simulink model "Studienarbeit"  (R2020a)
settings: Solver=VariableStepAuto  StartTime=0.0  StopTime=300  FixedStep=0.1  RelTol=1e-3
values from neighbouring files (symbols this model uses):
  driver_I = 0.1    [Buses_.mat]    (also in helperACCSetUp.m)
  driver_P = 0.2    [Buses_.mat]    (also in helperACCSetUp.m)
  initial_lane = 0    [helperACCSetUp.m]
  lr = 1.6    [Buses_.mat]    (also in helperACCSetUp.m)
  m = 1575    [Buses_.mat]    (also in helperACCSetUp.m)
  tau = 0.5    [Buses_.mat]    (also in helperACCSetUp.m)
  velocity_left_lane_max = 28    [Buses_.mat]    (also in helperManeuverSetUp.m)
  velocity_right_lane_max = 20    [Buses_.mat]    (also in helperManeuverSetUp.m)
  velocity_vehicle_B = 10    [Buses_.mat]    (also in helperManeuverSetUp.m)
  yawerr_gain = 2    [Buses_.mat]    (also in helperACCSetUp.m)
undefined symbols (not defined in the file or in its folder): Curvature, CurvatureDerivative, driving, HeadingAngle, LateralOffset, Left, Right, Strength
libraries: drivingscenarioandsensors x3, simulink x1, autolibshared x1
(part 2 of 2)

== matlab function Studienarbeit/Vehicle and Environment and Maneuver/Actors and Sensor Simulation/Pack Ego Actor ==
  data: pos input; egoActor output Bus: BusActors1Actors size=1; vel input; yaw input; yawRate input
function egoActor = packEgo(pos,vel,yaw,yawRate)
% Pack ego information into a single ego actor bus
%
% Imoprtant note:
% Output is a bus of type BusActorsActors. This is the same bus used by the
% Scenario Reader to output an individual actor. If you change the
% output bus name of Scenario Reader, change the output bus name here
% as well by clicking on 'Edit Data' in the menu above.
% if pos(2)<=-2
%     pos(2)=-2;
% elseif pos(2)>=2
%     pos(2)=2;
% end

egoActor = struct(...
    'ActorID',1,...
    'Position', [pos(1) pos(2) 0], ...
    'Velocity', [vel(1) vel(2) 0], ...
    'Roll', 0, ...
    'Pitch', 0, ...
    'Yaw', yaw, ...
    'AngularVelocity', [0 0 yawRate]);

== matlab function Studienarbeit/Vehicle and Environment and Maneuver/Control Unit/Steering Angle decide/Curve Lane or Not ==
  data: steeringLKA input; curve_lane_or_not output
function curve_lane_or_not = is_curve_lane(steeringLKA)
% This function uses steering angle from LKA to judge whether the lane 
% curve is,so that the vehicle will use another algorithm to achieve curve 
% lane changing.

% Input:
% steeringLKA: steering angle from Lane Keeping Assist.

% Output:
% curve_lane_or_not: 0->not a curve lane,1->curve lane.

if abs(steeringLKA) >10^(-2.5)%(-2.8)
    curve_lane_or_not = 1;
else
    curve_lane_or_not = 0;
end
% if abs(steeringLKA) >10^(-3)||(abs(Curvature_1)>10^(-4)||abs(Curvature_)>10^(-4))
%     curve_lane_or_not = 1;
% else
%     curve_lane_or_not = 0;
% end

== matlab function Studienarbeit/Vehicle and Environment and Maneuver/Control Unit/Steering Angle decide/Yaw Angle Process ==
  data: yaw_angle_ori input; yaw_angle output; curve_lane_or_not input
function yaw_angle = yaw_angle_process(yaw_angle_ori, curve_lane_or_not)
% This function subtracts a multiple of pi/2 rad from yaw angle when the 
% lane is straight,so that the vehicle can change its lane in straight lane 
% with a yaw angle larger than pi/2 rad.

% Inputs:
% yaw_angle_ori: original yaw angle(before processing).
% curve_lane_or_not: 0->not a curve lane,1->curve lane.

% Output:
% yaw_angle: the yaw angle after processing.

if curve_lane_or_not == 0
    yaw_angle=yaw_angle_ori-sign(yaw_angle_ori)*pi/2*round(abs(yaw_angle_ori)*2/pi);    
else 
    yaw_angle=yaw_angle_ori;
end

== stateflow chart Studienarbeit/Vehicle and Environment and Maneuver/Control Unit/Vehicle States ==
  state left_u_turn
    state decelerate
      entry:
      turn_flag = 5;
      coor_trans_t = clock_time;
      initial_lane_changing_velocity_ego = longitudinal_velocity;
    state turn_left
      entry:
      turn_flag = 6;
    state turn_left_1
      entry:
      turn_flag = 9;
    state backwards
      entry:
      turn_flag = 7;
    state turn_left_a_little
      entry:
      turn_flag = 8;
    decelerate -> turn_left : after(duration_lane_changing,sec)
    turn_left -> backwards : after(duration_lane_changing,sec)
    backwards -> turn_left_a_little : after(duration_lane_changing,sec)
    turn_left_a_little -> turn_left_1 : after(duration_lane_changing,sec)
  state switch_left_curve
    entry:
    turn_flag = 3;
  state switch_left
    entry:
    turn_flag = 1;
    coor_trans_t = clock_time;
    initial_lane_changing_velocity_ego = longitudinal_velocity;
  state lane_keeping
    entry:
    turn_flag = 0;
  state switch_right
    entry:
    turn_flag = 2;
    coor_trans_t = clock_time;
    initial_lane_changing_velocity_ego = longitudinal_velocity;
  state switch_right_curve
    entry:
    turn_flag = 4;
  note: command = 1, the vehicle switchs left,and turn_flag = 1.
      | command = 2, the vehicle switchs right,and turn_flag = 2.
      | if vehicle keeps lane, turn_flag = 0.
      | coor_trans_t is a time value which is used for coordinate transformation in
      | next subsystem:
      | "Duration,Curvature and Longitudinal Acceleration calculation".
      | initial_velocity_ego is the initial speed for the different maneuver.
      | current_lane = 0, the vehicle is at right lane.
      | current_lane = 1, the vehicle is at left lane
      | curve_lane_or_not = 0: the vehicle is driving at a curve lane.
      | curve_lane_or_not = 1: the vehicle is driving at a straight lane.
  lane_keeping -> decelerate [order 5] : [command == 5]
  lane_keeping -> switch_left_curve [order 3] : [command == 3]
  switch_left_curve -> lane_keeping : [left_boundary_strength>0.45&&right_boundary_strength< 0.15||left_lateral<0.22]{current_lane = 1;}
  (default) -> lane_keeping
  lane_keeping -> switch_left [order 2] : [command == 1]
  turn_left_1 -> lane_keeping : after(duration_lane_changing,sec){current_lane=1;}
  switch_left -> lane_keeping : after(duration_lane_changing,sec){current_lane = 1;}
  switch_right_curve -> lane_keeping : [left_boundary_strength<0.15&&right_boundary_strength >0.45||abs(right_lateral)<0.22]{current_lane = 0;}
  lane_keeping -> switch_right_curve [order 4] : [command==4]
  lane_keeping -> switch_right [order 1] : [command==2]
  switch_right -> lane_keeping : after(duration_lane_changing,sec){current_lane = 0;}
  data: turn_flag output; command input; clock_time input; coor_trans_t output; duration_lane_changing input; left_boundary_strength input; right_boundary_strength input; longitudinal_velocity input; initial_lane_changing_velocity_ego output; current_lane output; left_lateral input; right_lateral input
